simulink model "Backup"  (R2024b)
settings: Solver=ode3  StartTime=0  StopTime=TFinal  FixedStep=Ts  RelTol=1e-3  EnableMultiTasking=on
undefined symbols (not defined in the file): codertarget, Controller, DiscIntNeverNeededParam, Discrete, Estimator, g, gray, init, orient_ref, pos_ref, Sensors, Time, Ts, var_acc_angle_N, var_bias_gyr_N, var_gyro_p_N, Vehicle
libraries: simulink x52, matrix_library x5, slpidlib x4, ctrlSharedLib x4, sharedtransform x3, parrotlib x2
(part 3 of 3)

== stateflow chart Backup/Flight Control System/Path Planning/Chart1 ==
  state FindingLineLeft
    during:
    yawOut=yawOut-0.001;
  state TakeOff
    during:
    xout=0;
    yout=0;
    zout=-0.9;
    yawOut=0;
  state YawRight
    during:
    yawOut=yawOut+0.001;
    xout=xout+0.00035*cos(estim_YAW);
    yout=yout+0.00035*sin(estim_YAW);
  state MoveForward
    during:
    xout=xout+0.0005*cos(estim_YAW);
    yout=yout+0.0005*sin(estim_YAW);
  state YawLeft
    during:
    yawOut=yawOut-0.001;
    xout=xout+0.00035*cos(estim_YAW);
    yout=yout+0.00035*sin(estim_YAW);
  state FindingLineRight
    during:
    yawOut=yawOut+0.001
  state Land
    entry:
    zout=-0.1;
    landEnable = true;
  FindingLineLeft -> MoveForward : [up==1]
  TakeOff -> FindingLineLeft [order 1] : [after(3,sec)&&up==0&&LineLeft==1]
  (default) -> TakeOff
  YawRight -> MoveForward : [after(0.5,sec)&&up==1]
  TakeOff -> MoveForward [order 2] : [after(3,sec)&&up==1]
  MoveForward -> YawRight [order 1] : [right==1]
  TakeOff -> FindingLineRight [order 3] : [after(3,sec)&&up==0]
  YawLeft -> MoveForward : [after(0.5,sec)&&up==1]
  MoveForward -> YawLeft [order 2] : [left==1]
  FindingLineRight -> MoveForward : [up==1]
  MoveForward -> Land [order 3] : [circle==1&&right==0&&left==0]
  data: yawOut output single; xout output single; estim_YAW input; up input; circle input; left input; LineLeft input; yout output single; zout output single; landEnable output
